simulink library "speedgoatlib_fpga_pwm"  (R2024b)
settings: Solver=ode45  StartTime=0.0  StopTime=10.0  RelTol=1e-3  EnableMultiTasking=on
undefined symbols (not defined in the file): IO132, IO135, IO316, sg_fpga_callBackInit_m_a1, sg_fpga_cap_m_1
libraries: $bdroot x1
settings Model: Creator=dkraehenbuehl  LastModifiedBy=speedgoat\jenkins
settings SolverCC: AlgebraicLoopSolver=TrustRegion
settings DataIOCC: LimitDataPoints=on  ReturnWorkspaceOutputs=off
settings OptimizationCC: ReuseModelBlockBuffer=off  LifeSpan=inf
settings DebuggingCC: UnconnectedInputMsg=warning  UnconnectedOutputMsg=warning  UnconnectedLineMsg=warning  AllowSymbolicDim=off  PregeneratedLibrarySubsystemCodeDiagnostic=none  SFUnexpectedBacktrackingDiag=warning  SFNoUnconditionalDefaultTransitionDiag=warning  SFExecutionAtInitializationDiag=none  ArithmeticOperatorsInVariantConditions=warning
settings ModelReferenceCC: EnableRefExpFcnMdlSchedulingChecks=on
settings SFSimCC: SimUseLocalCustomCode=off  CustomCodeUndefinedFunction=UseInterfaceOnly
settings RTWCC: RTWUseLocalCustomCode=off  GPUComputeCapability=3.5  DLArmComputeVersion=19.05
settings CodeAppCC: StateflowObjectComments=on
settings GRTTargetCC: TargetLangStandard=C89/C90 (ANSI)
settings ConfigComp: CovMetricSettings=dw  CovSaveCumulativeToWorkspaceVar=on  CovSaveSingleToWorkspaceVar=on  CovExternalEMLEnable=off  CovBoundaryAbsTol=1.0e-5

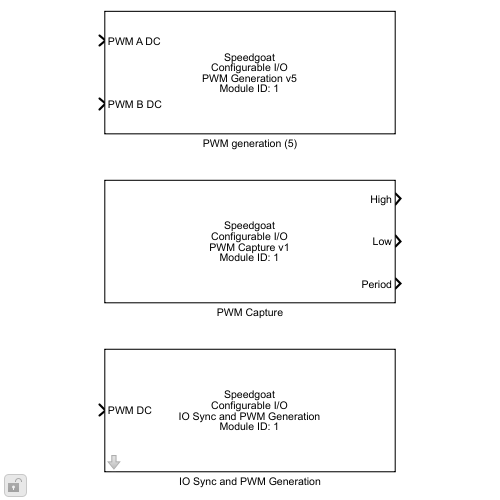
[thumbnail: Simulink's stored preview of the top-level diagram]
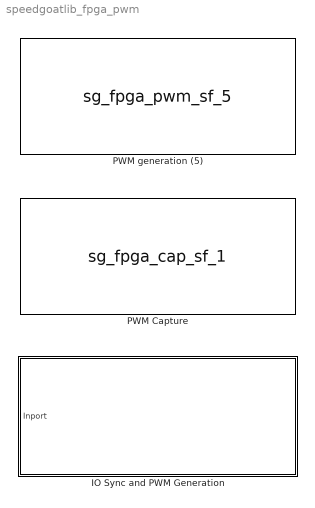
== system speedgoatlib_fpga_pwm ==
  IO Sync and PWM Generation : Subsystem  mask(Io_sync_and_pwm_generation){id=1, channelVector=[1:8], channelSelectionDropdown=1, ts=-1, basePwmPeriod=1e-3, actualBasePwmPeriod=1e-3, dutyCycleAlignment=Left-aligned, deadbandScalar=0, pwm_update=At period starts, ioModuleFamily=IO132-IO135, IO106_sampleMode=Multiple samples per period, IO106_Single_SamplePosition=Start of base PWM period, numberOfSamplesIO106=10, IO13x_sampleMode=Multiple samples per period, IO3x_Single_SamplePosition=Start of base PWM period, numberOfSamplesIO13x=10, IO13x_frameTriggerPosition=1, trigger_period_start=on, trigger_half_of_the_period=off, trigger_a_on=off, trigger_a_off=off, trigger_b_on=off, trigger_b_off=off}
      mask prompts: id "FPGA module identifier:"; channelVector "Channel vector:"; channelSelectionDropdown "Number of user PWM channels:"; ts "Sample time:"; basePwmPeriod "Desired base PWM period [s]"; actualBasePwmPeriod "Effective base PWM period [s]"; dutyCycleAlignment "Duty Cycle Alignement"; deadbandScalar "Deadband duration [s]"; pwm_update "Update PWM generation:"; ioModuleFamily "IO module family"; IO106_sampleMode "Sampling mode"; IO106_Single_SamplePosition "Sample position"; numberOfSamplesIO106 "Number of Samples per period"; IO13x_sampleMode "Sampling mode"; IO3x_Single_SamplePosition "Sample position"; numberOfSamplesIO13x "Number of samples per period"; IO13x_frameTriggerPosition "Frame trigger position"; trigger_period_start "Generate a trigger at period start"; trigger_half_of_the_period "Generate a trigger at half of the period"; trigger_a_on "Generate a trigger at A-On"; trigger_a_off "Generate a trigger at A-Off"; trigger_b_on "Generate a trigger at B-On"; trigger_b_off "Generate a trigger at B-Off"
      mask init:
      | sg_fpga_iosync_pwm_m();
      mask Help: eval('sg.utils.help.show(''io_main/refentry_io_sync_pwm_generation'');')
      mask TypeOptions id: PWM generation/id
      mask TypeOptions channelSelectionDropdown: 1 | 2 | 3 | 4 | 5 | 6 | 7 | 8 | 9 | 10 | 11 | 12 | 13 | 14 | 15 | 16
      mask TypeOptions ts: PWM generation/ts
      mask TypeOptions dutyCycleAlignment: SignalCalculation/dutyCycleAlignment
      mask TypeOptions pwm_update: PWM generation1/pwm_update
      mask TypeOptions ioModuleFamily: SignalCalculation/ioModuleFamily
      mask Callback ioModuleFamily:
      | ioModuleFamily = get_param(gcb, "ioModuleFamily");
      |     switch(ioModuleFamily)
      |         case 'IO106'
      |             %disp('Callback: IO106 case Mask Change');
      |             sg.mask.setControlVisible(gcb, 'Container13_IO13x', 'off');
      |             sg.mask.setControlVisible(gcb, 'Container12_IO106', 'on');
      |         case 'IO132-IO135'
      |             %disp('Callback: IO132-IO135 case Change');
      |             sg.mask.setControlVisible(gcb, 'Container13_IO13x', 'on');
      |             sg.mask.setControlVisible(gcb, 'Container12_IO106', 'off');
      |     end
      |     %disp(ioModuleFamily);
      mask TypeOptions IO106_sampleMode: Single sample per period | Multiple samples per period
      mask Callback IO106_sampleMode:
      | sampleMode = get_param(gcb, "IO106_sampleMode");
      |     switch(sampleMode)
      |         case 'Single sample per period'
      |             sg.mask.setControlVisible(gcb, 'Container12_IO106_Single', 'on');
      |             sg.mask.setControlVisible(gcb, 'Container13_IO106_Multiple', 'off');
      |         case 'Multiple samples per period'
      |              sg.mask.setControlVisible(gcb, 'Container12_IO106_Single', 'off');
      |             sg.mask.setControlVisible(gcb, 'Container13_IO106_Multiple', 'on');
      |     end
      mask TypeOptions IO106_Single_SamplePosition: Start of base PWM period | Middle of base PWM period
      mask TypeOptions IO13x_sampleMode: Single sample per period | Multiple samples per period
      mask Callback IO13x_sampleMode:
      | sampleMode = get_param(gcb, "IO13x_sampleMode");
      |     switch(sampleMode)
      |         case 'Single sample per period'
      |             sg.mask.setControlVisible(gcb, 'Container10_IO13x_Single', 'on');
      |             sg.mask.setControlVisible(gcb, 'Container10_IO13x_Multiple', 'off');
      |         case 'Multiple samples per period'
      |             sg.mask.setControlVisible(gcb, 'Container10_IO13x_Single', 'off');
      |             sg.mask.setControlVisible(gcb, 'Container10_IO13x_Multiple', 'on');
      |     end
      mask TypeOptions IO3x_Single_SamplePosition: Start of base PWM period | Middle of base PWM period
      mask TypeOptions trigger_period_start: PWM generation1/trigger_period_start
      mask TypeOptions trigger_half_of_the_period: PWM generation1/trigger_half_of_the_period
      mask TypeOptions trigger_a_on: PWM generation1/trigger_a_on
      mask TypeOptions trigger_a_off: PWM generation1/trigger_a_off
      mask TypeOptions trigger_b_on: PWM generation1/trigger_b_on
      mask TypeOptions trigger_b_off: PWM generation1/trigger_b_off
      mask DialogControl DescTextVar1 Prompt:
      | Speedgoat Driver Block
      | Configurable I/O - IO Sync and PWM Generation
      mask DialogControl DescTextVar2 Prompt: 2007 - 2026, Speedgoat GmbH
      mask DialogControl DescTextVar4 Prompt: www.speedgoat.com
      mask DialogControl Container5 Prompt: Module setup
      mask DialogControl channelNumberText1 Prompt: PWM CHANNEL INFORMATION
      mask DialogControl channelNumberText2 Prompt: Current synchronization format:                        IO132-IO135
      mask DialogControl channelNumberText3 Prompt: Sync PWM channels: 1, 2 - Conversion Clocks 3 - Frame Trigger
      mask DialogControl channelNumberText4 Prompt: PWM channels available to the user:                 4
      mask DialogControl channelNumberText5 Prompt: Total number of available PWM channels:          17
      mask DialogControl Container6 Prompt: PWM generation
      mask DialogControl Container11 Prompt: Intermodule Sync
      mask DialogControl IO106Text1 Prompt: SPEEDGOAT RECOMMENDATION: Based on your PWM period and sample settings, in the IO106 Analog input (DMA) block, select a Frame Size of 1, or a multiple thereof, to get a sample on every sample step, or every X sample steps, according to the selected multiple.
      mask DialogControl IO106Text2 Prompt: Timing Settings in IO106 Analog input (DMA) v2 block:
      mask DialogControl IO106Text3 Prompt: Inter-module Synchronization: Target
      mask DialogControl IO106Text4 Prompt: Frame Size: 10 or a multiple
      mask DialogControl IO106Text5 Prompt: ADC Clock [Hz] setting: 10000
      mask DialogControl IO106Text6 Prompt: For further information, refer to the speedgoat documentation.
      mask DialogControl IO13xText1 Prompt: SPEEDGOAT RECOMMENDATION: Based on your PWM period and sample settings, in the IO132-IO135 Setup block, enter following values:
      mask DialogControl IO13xText2 Prompt: Main tab:
      mask DialogControl IO13xText3 Prompt: Clock Base Rate: 20 MHz
      mask DialogControl IO13xText4 Prompt: Conversion clock divider: 2000
      mask DialogControl IO13xText4_aux Prompt: Conversio clock value might be rounded, caution when using the IO132-IO135 module as model trigger
      mask DialogControl IO13xText5 Prompt: 'Use Frame Trigger' check box: enabled
      mask DialogControl IO13xText6 Prompt: Frame Trigger Clock Divider: 10
      mask DialogControl IO13xText7 Prompt: Analog Inputs tab:
      mask DialogControl IO13xText8 Prompt: 'Enable DMA' check box: enabled
      mask DialogControl IO13xText9 Prompt: Frame Size (samples/channel): 10 or less
      mask DialogControl IO13xText10 Prompt: For further information, refer to the speedgoat documentation.
      mask DialogControl Container7 Prompt: Triggering
      mask Display: disp('Speedgoat\nConfigurable I/O\nIO Sync and PWM Generation\nModule ID: 1');port_label('input',1,'PWM DC');
  PWM Capture : S-Function  InitFcn=sg_fpga_cap_m_1.runInitFcn()  FunctionName=sg_fpga_cap_sf_1  Parameters=fpgaFrequency, id, chan, showHighDuration, showLowDuration, showDC16, showDC8, showTOn, showTOff, showPeriod, showValidData, captureMode, captureTimeout_si, ts, debounce_si  SFunctionDeploymentMode=off  EnableBusSupport=off  mask(cap_fpga_1){id=1, chan=[1], ts=0.001, captureMode=High transitions triggered, bit_width_cap=24, captureTimeout_si=0, captureTimeout_eff=[0], debounce_si=100e-9, debounce_eff=[106.7e-9], showHighDuration=on, showLowDuration=on, showPeriod=on, showDC16=off, showDC8=off, showTOn=off, showTOff=off, showValidData=off}
      mask prompts: id "Configurable I/O Module ID"; chan "Channel vector:"; ts "Sample time:"; captureMode "Capture mode:"; bit_width_cap "Bit width CAP measurement"; captureTimeout_si "Capture timeout vector [s]:"; captureTimeout_eff "Effective capture timeout [s]"; debounce_si "Debounce time vector [s]"; debounce_eff "Effective debounce time [s]"; showHighDuration "Show high duration"; showLowDuration "Show low duration"; showPeriod "Show period"; showDC16 "Show duty cycle (16 bits)"; showDC8 "Show duty cycle (8 bits)"; showTOn "Show TOn"; showTOff "Show TOff"; showValidData "Show Valid Data Flag"
      mask help: Speedgoat Driver Block<br>Configurable I/O - PWM Capture<br><br>&copy; 2007 - 2026, Speedgoat GmbH, <a href="matlab: web('www.speedgoat.com','-browser');">www.speedgoat.com</a>
      mask init:
      | fpgaFrequency = NaN;
      | [fpgaFrequency, debounce_si, captureMode, captureTimeout_si] = sg_fpga_cap_m_1.runMaskInit();
      mask Help: eval('sg.utils.help.show(''io_main/refentry_pwm_capture_v1'');')
      mask TypeOptions id: 1 | 2 | 3 | 4 | 5 | 6 | 7 | 8 | 9 | 10
      mask TypeOptions captureMode: High transitions triggered | Low transitions triggered | Use dedicated trigger input | Software triggered
      mask Callback captureTimeout_si: %sg_fpga_cap_m_1('captureTimeout_si');
      mask Callback debounce_si: %sg_fpga_cap_m_1('debounce_si');
      mask DialogControl ParameterTabVar0 Prompt: Module setup
      mask DialogControl ParameterTabVar01 Prompt: Capture
      mask DialogControl TimeoutContainer Prompt: Capture Timeout
      mask DialogControl debounceContainer Prompt: Channel debounce time
      mask DialogControl ParameterTabVar012 Prompt: Input and output port configuration
      mask Display: disp('Speedgoat\nConfigurable I/O\nPWM Capture v1\nModule ID: 1');port_label('output',1,'High');port_label('output',2,'Low');port_label('output',3,'Period');
  PWM generation (5) : S-Function  InitFcn=sg_fpga_callBackInit_m_a1;  FunctionName=sg_fpga_pwm_sf_5  Parameters=id, chan, fpga_frequency, symmetric, invert_a, invert_b, invert_c, bit_width_pwm_gen, period, a_on, a_off, b_on, b_off, c_on, c_off, trigger_duration, protection, enable_latch_half_period, trigger_source, idle_a, idle_b, idle_c, deadband, show_a_input, show_b_input, show_c_input, show_period_input, b_is_complement_of_a, pwm_a_dc, pwm_b_dc, show_force_stop_input, cancels_pwm_generation, delay, enable_natural_pwm, ts  SFunctionDeploymentMode=off  EnableBusSupport=off  mask(pwm_fpga_5){id=1, chan=[1], board=Please select..., ts=0.001, pciSlot=-1, delay=0, symmetric=Symmetric - PWM generation is centered around half the period, b_is_complement_of_a=Independent of PWM A output, deadband=[0.0], period=0.001, frequency=1000, ticks=74999, a_on=[0], a_off=[0], pwm_a_dc=[0.0], b_on=[0], b_off=[0], pwm_b_dc=[0], c_on=[0.0], c_off=[0.0], protection=Disabled: A and B can be high at the same moment, enable_latch_half_period=off, pwm_update=At period starts, bit_width_pwm_gen=24, trigger_duration=[1e-6], trigger_period_start=off, trigger_half_of_the_period=off, trigger_a_on=off, trigger_a_off=off, trigger_b_on=off, trigger_b_off=off, show_a_input=on, show_b_input=on, show_c_input=off, show_period_input=off, show_force_stop_input=off, idle_a=Low when PWM generation is halted, idle_b=Low when PWM generation is halted, idle_c=Low when PWM generation is halted, cancels_pwm_generation=on, invert_a=off, invert_b=off, invert_c=off}
      mask prompts: id "Configurable I/O Module ID"; chan "Channel vector:"; ts "Sample time:"; pciSlot "PCI slot (-1: autosearch):"; delay "PWM phase vector [s]:"; symmetric "PWM pattern is:"; b_is_complement_of_a "PWM B output is:"; deadband "Deadband duration vector [s]:"; period "Initial period vector [s]:"; frequency "Initial frequency vector [Hz]:"; ticks "Number of Ticks"; a_on "Initial A-On vector [s]:"; a_off "Initial A-Off vector [s]:"; pwm_a_dc "Initial PWM A duty cycle vector:"; b_on "Initial B-On vector [s]:"; b_off "Initial B-Off vector [s]:"; pwm_b_dc "Initial PWM B duty cycle vector:"; c_on "Initial C-On vector [s]:"; c_off "Initial C-Off vector [s]:"; protection "AB-output protection:"; enable_latch_half_period "Enable the second update at half of PWM period"; pwm_update "Update PWM generation:"; bit_width_pwm_gen "Bit width PWM generation"; trigger_duration "Trigger duration vector [s]:"; trigger_period_start "Generate a trigger at period start"; trigger_half_of_the_period "Generate a trigger at half of the period"; trigger_a_on "Generate a trigger at A-On"; trigger_a_off "Generate a trigger at A-Off"; trigger_b_on "Generate a trigger at B-On"; trigger_b_off "Generate a trigger at B-Off"; show_a_input "Show A input port"; show_b_input "Show B input port"; show_c_input "Show C input port"; show_period_input "Show period input port"; show_force_stop_input "Show PWM generation halt input port"; idle_a "PWM output A is:"; idle_b "PWM output B is:"; idle_c "PWM output C/Trigger is:"; cancels_pwm_generation "When model stops, PWM Generation halts after completion of PWM period"; invert_a "Invert A output"; invert_b "Invert B output"; invert_c "Invert C/Trigger output"
      mask help: Speedgoat Driver Block<br>Configurable I/O - PWM Generation<br><br>&copy; 2007 - 2026, Speedgoat GmbH, <a href="matlab: web('www.speedgoat.com','-browser');">www.speedgoat.com</a>
      mask init:
      | fpga_frequency = NaN;
      | 
      | [fpga_frequency, period, a_on, a_off, b_on, b_off, c_on, c_off, invert_a, invert_b, invert_c, ...
      |  idle_a, idle_b, idle_c, trigger_duration, protection, enable_latch_half_period, deadband, trigger_source, ...
      |  b_is_complement_of_a, show_b_input, pwm_a_dc, pwm_b_dc, cancels_pwm_generation, delay, enable_natural_pwm] ...
      |  = sg_fpga_pwm_m_5();
      mask Help: eval('sg.utils.help.show(''io_main/refentry_pwm_generation_v5'');')
      mask TypeOptions id: 1 | 2 | 3 | 4 | 5 | 6 | 7 | 8 | 9 | 10
      mask TypeOptions symmetric: Symmetric - PWM generation is centered around half the period | Asymmetric - On and Off are freely configurable
      mask Callback symmetric: sg_fpga_pwm_m_5_display('calback_symmetric');
      mask TypeOptions b_is_complement_of_a: The complement of PWM A output | Independent of PWM A output
      mask Callback b_is_complement_of_a: sg_fpga_pwm_m_5_display('calback_b_is_complement_of_a');
      mask Callback period: sg_fpga_pwm_m_5_display('callback_period');
      mask Callback frequency: %sg_fpga_pwm_m_5_display('callback_frequency');
      mask TypeOptions protection: Disabled: A and B can be high at the same moment | A is forced off when B is on. | B is forced off when A is on. | A/B are forced off when A/B are on.
      mask TypeOptions pwm_update: At period starts | At period starts and at half of the PWM period | Always (natural PWM update)
      mask TypeOptions idle_a: Low when PWM generation is halted | High when PWM generation is halted
      mask TypeOptions idle_b: Low when PWM generation is halted | High when PWM generation is halted
      mask TypeOptions idle_c: Low when PWM generation is halted | High when PWM generation is halted
      mask DialogControl Container4 Prompt: Module setup
      mask DialogControl Container5 Prompt: PWM generation
      mask DialogControl Container8 Prompt: Triggering
      mask DialogControl Container10 Prompt: Input ports configuration
      mask DialogControl Container7 Prompt: Offline state
      mask DialogControl Container14 Prompt: Polarity
      mask Display: disp('Speedgoat\nConfigurable I/O\nPWM Generation v5\nModule ID: 1');port_label('input',1,'PWM A DC');port_label('input',2,'PWM B DC');

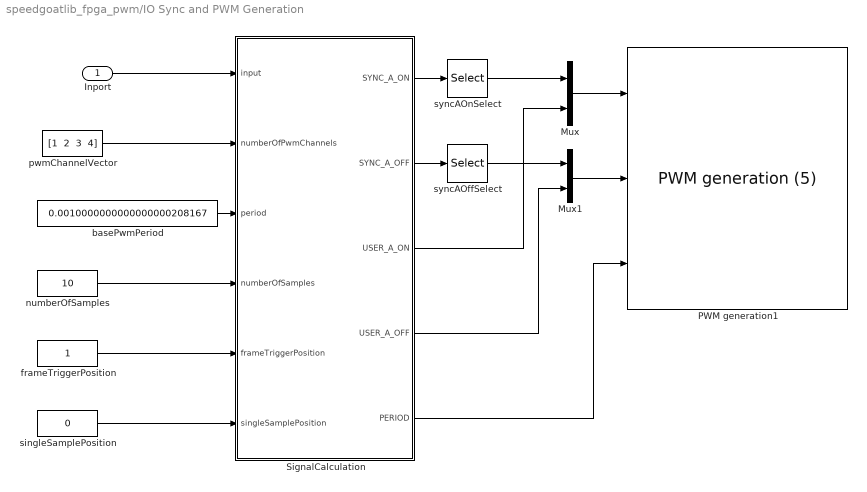
== system speedgoatlib_fpga_pwm/IO Sync and PWM Generation ==
  Inport : Inport  PortDimensions=1
  Mux : Mux  Inputs=2
  Mux1 : Mux  Inputs=2
  PWM generation1 : $bdroot/PWM generation (5)  id=1  chan="[1  2  3  4]"  board=IO316-100k  ts=ts  pciSlot=[-1,-1]  delay=0  symmetric=Asymmetric - On and Off are freely configurable  b_is_complement_of_a=The complement of PWM A output  deadband=0  period=0  frequency=Inf  ticks=-1  a_on=0  a_off=0  pwm_a_dc=[0.0]  b_on=[0]  b_off=[0]  pwm_b_dc=[0]  c_on=[0.0]  c_off=[0.0]  protection=Disabled: A and B can be high at the same moment  enable_latch_half_period=off  pwm_update=At period starts  bit_width_pwm_gen=24  trigger_duration=[1e-6]  trigger_period_start=on  trigger_half_of_the_period=off  trigger_a_on=off  trigger_a_off=off  trigger_b_on=off  trigger_b_off=off  show_a_input=on  show_b_input=on  show_c_input=off  show_period_input=on  show_force_stop_input=off  idle_a=High when PWM generation is halted  idle_b=Low when PWM generation is halted  idle_c=Low when PWM generation is halted  cancels_pwm_generation=off  invert_a=off  invert_b=off  invert_c=off
  SignalCalculation : MATLAB Function  TreatAsAtomicUnit=on  mask{ioModuleFamily=IO132-IO135, dutyCycleAlignment=Left-aligned}
      mask prompts: ioModuleFamily "IO module family"; dutyCycleAlignment "Duty Cycle Alignement"
  basePwmPeriod : Constant  Value=0.0010000000000000000208167
  frameTriggerPosition : Constant
  numberOfSamples : Constant  Value=10
  pwmChannelVector : Constant  Value="[1  2  3  4]"
  singleSamplePosition : Constant  Value=0
  syncAOffSelect : Selector  InputPortWidth=3  IndexOptions=Index vector (dialog)  Indices=1:3  OutputSizes=1
  syncAOnSelect : Selector  InputPortWidth=3  IndexOptions=Index vector (dialog)  Indices=1:3  OutputSizes=1
  wires:
  singleSamplePosition/1 -> SignalCalculation/6(singleSamplePosition)
  Inport/1 -> SignalCalculation/1(input)
  basePwmPeriod/1 -> SignalCalculation/3(period)
  numberOfSamples/1 -> SignalCalculation/4(numberOfSamples)
  frameTriggerPosition/1 -> SignalCalculation/5(frameTriggerPosition)
  pwmChannelVector/1 -> SignalCalculation/2(numberOfPwmChannels)
  SignalCalculation/5(PERIOD) -> PWM generation1/3
  Mux/1 -> PWM generation1/1
  SignalCalculation/3(USER_A_ON) -> Mux/2
  SignalCalculation/4(USER_A_OFF) -> Mux1/2
  SignalCalculation/2(SYNC_A_OFF) -> syncAOffSelect/1
  Mux1/1 -> PWM generation1/2
  SignalCalculation/1(SYNC_A_ON) -> syncAOnSelect/1
  syncAOnSelect/1 -> Mux/1
  syncAOffSelect/1 -> Mux1/1

== matlab function speedgoatlib_fpga_pwm/IO Sync and PWM Generation/SignalCalculation ==
  data: SYNC_A_ON output; SYNC_A_OFF output; input input; numberOfPwmChannels input; period input; USER_A_ON output; USER_A_OFF output; PERIOD output; numberOfSamples input; frameTriggerPosition input; singleSamplePosition input; ioModuleFamily parameter; dutyCycleAlignment parameter
function [SYNC_A_ON, SYNC_A_OFF, USER_A_ON, USER_A_OFF, PERIOD]= fcn(input, numberOfPwmChannels, period, numberOfSamples,frameTriggerPosition, singleSamplePosition, ioModuleFamily, dutyCycleAlignment)
    %Initialize array sizes
    numberOfPwmChannels = length(numberOfPwmChannels);
    for i=1:length(input)
        if input(i) < 0
            input(i) = 0;
        elseif input(i) > 1
            input(i) = 1;
        end
    end
    %SYNC_A_ON106 = zeros(3,1);
    %SYNC_A_OFF106 = zeros(3,1);
    %SYNC_A_ON13x = zeros(3,1);
    %SYNC_A_OFF13x = zeros(3,1);
    SYNC_A_ON = zeros(3,1);
    SYNC_A_OFF = zeros(3,1);
    USER_A_ON = zeros((length(input)),1);
    USER_A_OFF = zeros((length(input)),1);

    switch(dutyCycleAlignment)
        case 1 % 'Center-aligned'
            for i = 1:(length(USER_A_ON))
                USER_A_ON(i)    = (period/2)-(period*input(i))/2; 
                USER_A_OFF(i)   = (period/2)+(period*input(i))/2;
            end
        case 2 % 'Left-aligned'
            for i = 1:(length(USER_A_ON))
                USER_A_ON(i)    = 0;
                USER_A_OFF(i)   = period*input(i);
            end
        case 3 % 'Right-aligned'
            for i = 1:(length(USER_A_ON))
                if input(i) < (1-1e-7) % NOTE: to avoid PWM beeing zero all the time when DC is almost 1
                    USER_A_ON(i)    = period*(1-input(i));
                    USER_A_OFF(i)   = 0;
                else
                    USER_A_ON(i)    = 0;
                    USER_A_OFF(i)   = period;
                end
            end
    end
    

    PERIOD = ones((numberOfPwmChannels),1)*period;
    tAdc        = 0;
    adcTon      = 0;
    adcToff     = 0;
    fTrigTon    = 0;
    fTrigToff   = 0;

    %Check which module Family
    switch(ioModuleFamily)
        case 1 % 'IO106'
            if numberOfSamples > 1
                %Multiple samples per frame
                %ADC Clock Signal
                adcTon  = 1e-6;
                adcToff = 0;
                PERIOD(1) = period/numberOfSamples;
                %Todo: Adapt Period Base PWM Period / Number of Samples
            else
                %Single sample per frame
                %check sample position
                switch(singleSamplePosition)
                    case 1 %start of base PWM period
                        %ADC Clock Signal
                        adcTon  = 1e-6;
                        adcToff = 0;
                        %Period size == Base PWM Period
                    case 2 %middle of base PWM period
                        %ADC Clock Signal
                        adcTon  = (period/2)+1e-6;
                        adcToff = period/2;
                        %Period size == Base PWM Period
                end
            end
            %ADC Sync signal
            SYNC_A_ON(1)    = adcTon;
            SYNC_A_OFF(1)   = adcToff;
            

        case 2 % 'IO132-IO135'

            if numberOfSamples > 1
                %Multiple samples per frame
                %ADC Clock Signal
                tAdc = period/numberOfSamples;
                adcTon = tAdc/2;
                adcToff = 0;
                %Frame Trigger Signal
                fTrigTon = tAdc*frameTriggerPosition;
                fTrigToff = tAdc*(frameTriggerPosition-0.5);
                PERIOD(1) = period/numberOfSamples;
                PERIOD(2) = period/numberOfSamples;
            else
                %Single sample per frame
                %check sample position
                switch(singleSamplePosition)
                    case 1 %start of base PWM period
                        %ADC Clock Signal
                        adcTon      = 2.5e-6;
                        adcToff     = 0;
                        %Frame Trigger Signal
                        fTrigTon    = 5e-6;
                        fTrigToff   = 2.5e-6;
                    case 2 %middle of base PWM period
                        %ADC Clock Signal
                        adcTon      = (period/2)+2.5e-6;
                        adcToff     = period/2;
                        %Frame Trigger Signal
                        fTrigTon    = (period/2)+5e-6;
                        fTrigToff   = (period/2)+2.5e-6;
                end
            end
            %Conversion clock 1
            SYNC_A_ON(1)    = adcTon;
            SYNC_A_OFF(1)   = adcToff;
            %Conversion clock 2
            SYNC_A_ON(2)    = adcTon;
            SYNC_A_OFF(2)   = adcToff;
            %Frame Trigger Signal
            SYNC_A_ON(3)    = fTrigTon;
            SYNC_A_OFF(3)   = fTrigToff;
    end
end
